simulink model "ERR_H3"  (R2025a)
settings: Solver=VariableStepAuto  StartTime=0.0  StopTime=50  MaxStep=1/50  RelTol=1e-3
InitFcn:
  | % Állandósult állapoti erősítés
  | K = 5;
  | 
  | % Időállandó
  | tau = 2.5;      % s
settings Model: Creator=Szalay  LastModifiedBy=Szalay

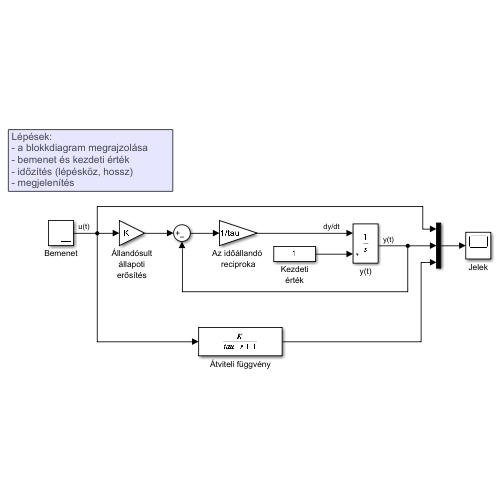
[thumbnail: Simulink's stored preview of the top-level diagram]
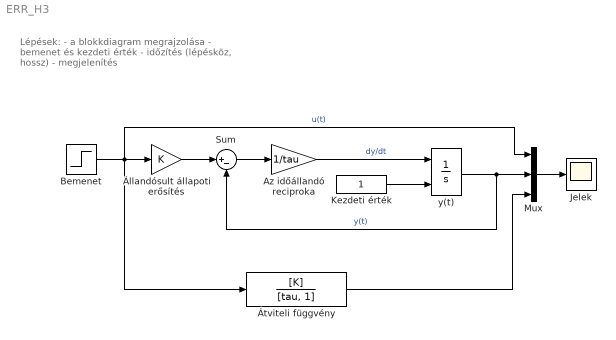
== system ERR_H3 ==
  note: Lépések:
      | - a blokkdiagram megrajzolása
      | - bemenet és kezdeti érték
      | - időzítés (lépésköz, hossz)
      | - megjelenítés
  Az időállandó reciproka : Gain  Gain=1/tau
  Bemenet : Step  Time=0  After=-2  SampleTime=0
  Jelek : Scope
      settings: ActiveDisplayYMinimum=-0.18668058593539105  ActiveDisplayYMaximum=1.0735733206443165
  Kezdeti érték : Constant
  Mux : Mux  Inputs=3
  Sum : Sum  Inputs=|+-
  y(t) : Integrator  InitialConditionSource=external
  Állandósult állapoti erősítés : Gain  Gain=K
  Átviteli függvény : TransferFcn  Numerator=[K]  Denominator=[tau, 1]
  wires:
  Az időállandó reciproka/1 -> y(t)/1  "dy/dt"
  Sum/1 -> Az időállandó reciproka/1
  y(t)/1 -> Sum/2, Mux/2  "y(t)"
  Állandósult állapoti erősítés/1 -> Sum/1
  Bemenet/1 -> Átviteli függvény/1, Mux/1, Állandósult állapoti erősítés/1  "u(t)"
  Kezdeti érték/1 -> y(t)/2
  Mux/1 -> Jelek/1
  Átviteli függvény/1 -> Mux/3
